simulink model "pendulum_plant"  (R2018b)
settings: Solver=VariableStepAuto  StartTime=0.0  StopTime=10.0  RelTol=1e-3
values from neighbouring files (symbols this model uses):
  g = 9.8    [inverted_pendulum.m]    (also in inverted_pendulum_final.m)
undefined symbols (not defined in the file or in its folder): lp
settings Model: Creator=ipebo  LastModifiedBy=ipebo

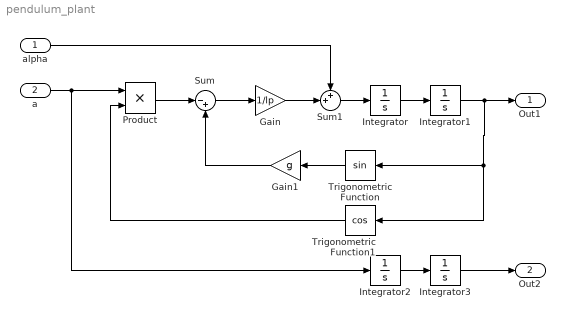
== system pendulum_plant ==
  alpha : Inport
  a : Inport  Port=2
  Gain : Gain  Gain=1/lp
  Gain1 : Gain  Gain=g
  Integrator{,1..3} (4 alike) : Integrator
  Product : Product
  Sum : Sum  Inputs=|-+
  Sum1 : Sum  Inputs=++|
  Trigonometric Function : Trigonometry
  Trigonometric Function1 : Trigonometry  Operator=cos
  Out1 : Outport  SignalName=theta
  Out2 : Outport  Port=2  SignalName=s
  wires:
  a/1 -> Integrator2/1, Product/1
  Product/1 -> Sum/1
  Sum/1 -> Gain/1
  Sum1/1 -> Integrator/1
  Integrator/1 -> Integrator1/1
  Integrator1/1 -> Out1/1, Trigonometric Function1/1, Trigonometric Function/1
  Trigonometric Function/1 -> Gain1/1
  Gain1/1 -> Sum/2
  alpha/1 -> Sum1/1
  Gain/1 -> Sum1/2
  Trigonometric Function1/1 -> Product/2
  Integrator2/1 -> Integrator3/1
  Integrator3/1 -> Out2/1
